simulink model "delay_planta3"  (Simulink 6.0)
settings: Solver=ode45  StartTime=0.0  StopTime=10.0  RelTol=1e-3
settings Model: LastModifiedBy=JaPa

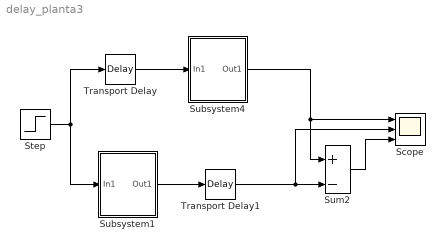
== system delay_planta3 ==
  Scope : Scope  NumInputPorts=3
      settings: AttributesFormatString=%<BackgroundColor>  TimeRange=10  YMin=0.5~0.5~-1  YMax=4~4~4
  Step : Step  Time=0  SampleTime=0
  Subsystem1 : Subsystem
      mask Display: disp('Planta P3')
  Subsystem4 : Subsystem
      mask Display: disp('Planta P3')
  Sum2 : Sum  Inputs=|+-
  Transport Delay : TransportDelay  DelayTime=3
  Transport Delay1 : TransportDelay  DelayTime=3
  wires:
  Transport Delay/1 -> Subsystem4/1(In1)
  Subsystem1/1(Out1) -> Transport Delay1/1
  Subsystem4/1(Out1) -> Scope/1, Sum2/1
  Transport Delay1/1 -> Scope/2, Sum2/2
  Sum2/1 -> Scope/3
  Step/1 -> Transport Delay/1, Subsystem1/1(In1)

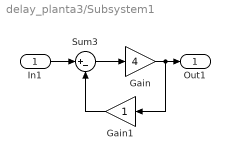
== system delay_planta3/Subsystem1 ==
  In1 : Inport  Port=1  LatchInput=off
  Gain : Gain  Gain=4
  Gain1 : Gain  Orientation=left
  Sum3 : Sum  Inputs=|+-
  Out1 : Outport
  wires:
  Sum3/1 -> Gain/1
  Gain1/1 -> Sum3/2
  Gain/1 -> Out1/1, Gain1/1
  In1/1 -> Sum3/1

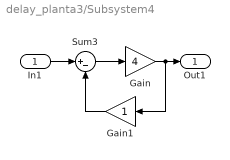
== system delay_planta3/Subsystem4 ==
  In1 : Inport  Port=1  LatchInput=off
  Gain : Gain  Gain=4
  Gain1 : Gain  Orientation=left
  Sum3 : Sum  Inputs=|+-
  Out1 : Outport
  wires:
  In1/1 -> Sum3/1
  Gain/1 -> Gain1/1, Out1/1
  Gain1/1 -> Sum3/2
  Sum3/1 -> Gain/1
